simulink model "COMPose"  (Simulink 7.9)
settings: Solver=ode45  StartTime=0.0  StopTime=inf  FixedStep=1  RelTol=1e-3
libraries: utility x1, dspmtrx3 x1, simulink x1
settings Model: Creator=jorhabib  LastModifiedBy=jorhabib

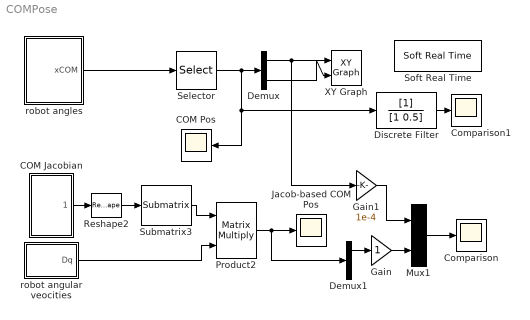
== system COMPose ==
  COM Jacobian : Subsystem
  COM Pos : Scope
      settings: TimeRange=200  YMin=-0.07  YMax=0.07  SampleTime=0.02
  Comparison : Scope
      settings: TickLabels=on  TimeRange=10  YMin=2.11758e-22  YMax=6e-06  SampleTime=0.02
  Comparison1 : Scope
      settings: TickLabels=on  TimeRange=50  YMin=-0.05  YMax=0.05  SampleTime=0.02
  Demux : Demux  Outputs=2
  Demux1 : Demux  Outputs=2
  Discrete Filter : DiscreteFilter  SampleTime=0.02
  Gain : Gain
  Gain1 : Gain  Gain=1e-4
  Jacob-based COM Pos : Scope
      settings: TimeRange=10  YMin=-8.999999999999999e-06  YMax=8.999999999999999e-06  SaveName=ScopeData4  SampleTime=0.02
  Mux1 : Mux  Inputs=2
  Product2 : Product  Multiplication=Matrix(*)  RndMeth=Zero
  Reshape2 : Reshape  OutputDimensionality=Customize  OutputDimensions=[6,31]
  Selector : Selector  InputPortWidth=7  IndexOptions=Index vector (dialog)  Indices=[1:2]  OutputSizes=1
  Soft Real Time : utility/Soft Real Time  x=0.020
  Submatrix3 : dspmtrx3/Submatrix  RowSpan=Range of rows  RowStartMode=First  RowStartIndex=1  RowEndMode=Index  RowEndIndex=2  ColSpan=Range of columns  ColStartMode=Index  ColStartIndex=7  ColEndMode=Last  ColEndIndex=6
  XY Graph : simulink/Sinks/XY Graph  xmin=-0.1  xmax=0.01  ymin=-0.05  ymax=0.05  st=-1
  robot angles : Subsystem
  robot angular veocities : Subsystem
  wires:
  robot angles/1(xCOM) -> Selector/1
  Selector/1 -> Demux/1, COM Pos/1, Discrete Filter/1
  Demux/2 -> XY Graph/1
  Demux/1 -> XY Graph/2, Gain1/1
  COM Jacobian/1(Jacobian) -> Reshape2/1
  Reshape2/1 -> Submatrix3/1
  Submatrix3/1 -> Product2/1
  robot angular veocities/1(Dq) -> Product2/2
  Product2/1 -> Jacob-based COM Pos/1, Demux1/1
  Mux1/1 -> Comparison/1
  Demux1/1 -> Gain/1
  Gain/1 -> Mux1/2
  Gain1/1 -> Mux1/1
  Discrete Filter/1 -> Comparison1/1

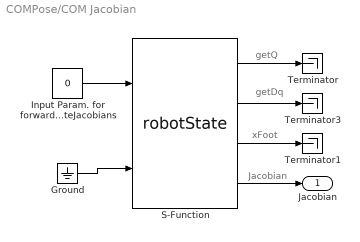
== system COMPose/COM Jacobian ==
  note: getDq
  note: xFoot
  note: getQ
  note: Jacobian
  Ground : Ground
  "Input Param. for forwardKinematics and  computeJacobians " : Constant  Value=0  OutDataTypeStr=int8
  S-Function : S-Function  FunctionName=robotState  Parameters=val,robotname,localname  EnableBusSupport=off  mask{val=3, robotname='icubSim', localname='robotState'}
      mask prompts: val "Value"; robotname "Robot Name (icub - icubSim)"; localname "Module Name"
  Terminator : Terminator
  Terminator1 : Terminator
  Terminator3 : Terminator
  Jacobian : Outport
  wires:
  Ground/1 -> S-Function/2
  S-Function/2 -> Terminator3/1
  S-Function/1 -> Terminator/1
  S-Function/3 -> Terminator1/1
  "Input Param. for forwardKinematics and  computeJacobians "/1 -> S-Function/1
  S-Function/4 -> Jacobian/1

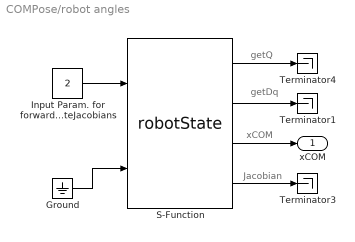
== system COMPose/robot angles ==
  note: Jacobian
  note: getQ
  note: xCOM
  note: getDq
  Ground : Ground
  "Input Param. for forwardKinematics and  computeJacobians " : Constant  Value=2  OutDataTypeStr=int8
  S-Function : S-Function  FunctionName=robotState  Parameters=val,robotname,localname  EnableBusSupport=off  mask{val=2, robotname='icubSim', localname='robotState'}
      mask prompts: val "Value"; robotname "Robot Name (icub - icubSim)"; localname "Module Name"
  Terminator1 : Terminator
  Terminator3 : Terminator
  Terminator4 : Terminator
  xCOM : Outport
  wires:
  S-Function/4 -> Terminator3/1
  "Input Param. for forwardKinematics and  computeJacobians "/1 -> S-Function/1
  S-Function/3 -> xCOM/1
  S-Function/1 -> Terminator4/1
  S-Function/2 -> Terminator1/1
  Ground/1 -> S-Function/2

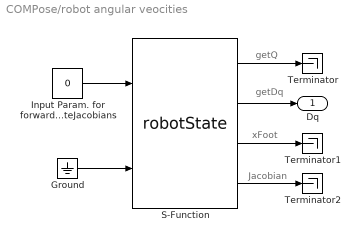
== system COMPose/robot angular veocities ==
  note: getDq
  note: xFoot
  note: getQ
  note: Jacobian
  Ground : Ground
  "Input Param. for forwardKinematics and  computeJacobians " : Constant  Value=0  OutDataTypeStr=int8
  S-Function : S-Function  FunctionName=robotState  Parameters=val,robotname,localname  EnableBusSupport=off  mask{val=1, robotname='icubSim', localname='robotState'}
      mask prompts: val "Value"; robotname "Robot Name (icub - icubSim)"; localname "Module Name"
  Terminator : Terminator
  Terminator1 : Terminator
  Terminator2 : Terminator
  Dq : Outport
  wires:
  Ground/1 -> S-Function/2
  S-Function/2 -> Dq/1
  S-Function/1 -> Terminator/1
  S-Function/3 -> Terminator1/1
  "Input Param. for forwardKinematics and  computeJacobians "/1 -> S-Function/1
  S-Function/4 -> Terminator2/1
